simulink model "sampleModel255"  (R2021b)
settings: Solver=VariableStepAuto  StartTime=0.0  StopTime=10.0  RelTol=1e-3
undefined symbols (not defined in the file or in its folder): Newton, Raphson
libraries: simulink x14, slpidlib x3
settings Model: Creator=user  LastModifiedBy=user

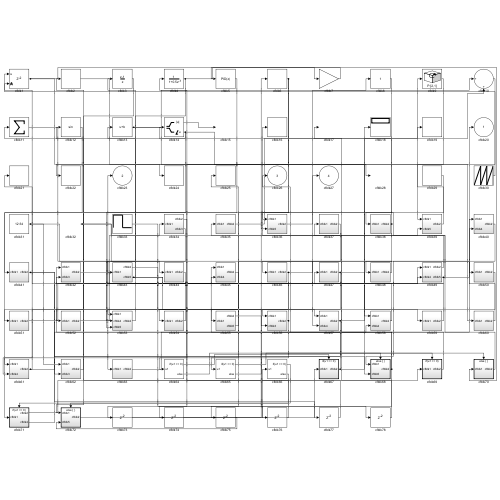
[thumbnail: Simulink's stored preview of the top-level diagram]
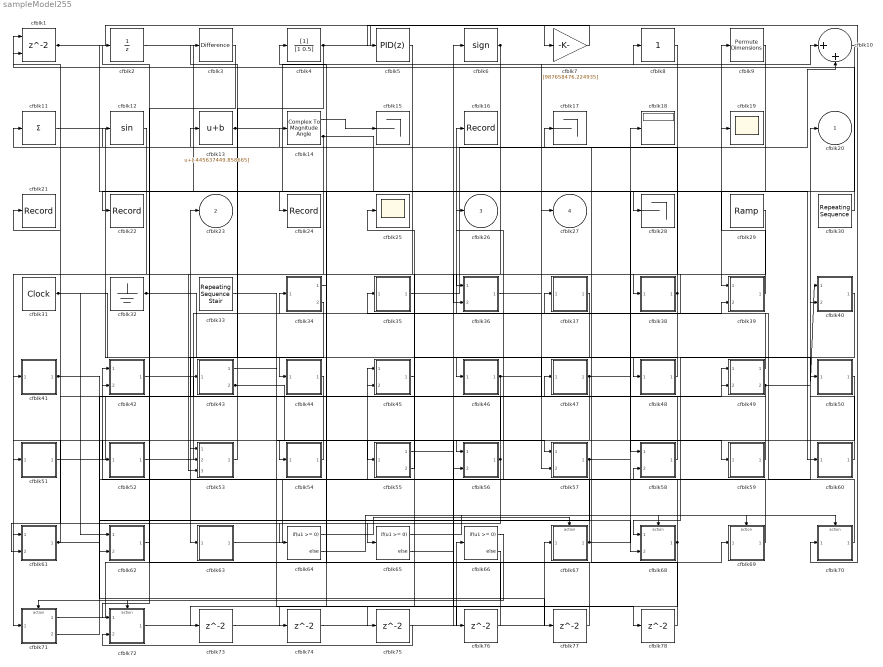
== system sampleModel255 ==
  cfblk1 : Delay  ShowEnablePort=on  SampleTime=1
      settings: InputPortMap=u0,e6
  cfblk10 : Sum  Inputs=|++
  cfblk11 : Sum  Inputs=+
  cfblk12 : Trigonometry
  cfblk13 : Bias  Bias=[-445637449.858665]
  cfblk14 : ComplexToMagnitudeAngle
  cfblk15 : Terminator
  cfblk16 : Record  FileSettingsInternal="{\"entries\":[{\"content\":{\"excelSettings\":{\"content\":{},\"type\":\"Streamout.ExcelSettings\"}},\"type\":\"Streamout.FileSettingStorage\",\"uuid\":\"bcba30e2-a7e8-405a-9570-f6df06466bcb\"}],\"packageUris\":[\"http://schema.mathworks.com/mf0/streamout_blocks/R2020a\"],\"version\":\"1.0\"}"  SignalsInternal="{\"entries\":[{\"content\":{\"signals\":[{\"content\":{\"blockPath\":[\"sampleModel255/cfblk16\"],\"channel\":[],\"dimensions\":[1],\"domain\":\"sampleModel255/cfblk16\",\"lineColor\":\"#a2142f\",\"plots\":[1],\"port\":1,\"sid\":[\"\"],\"signalID\":10495,\"signalName\":\"cfblk49:1\"},\"type\":\"RecordBlkView.Signal\",\"uuid\":\"f066bb72-dd2c-4bd8-bcfc-d20f2ea079be\"}]},\"type\":\"RecordBlkView.InputSignals\",\"uuid\":\"8c248f1a-7e81-44ad-9cf1-3fb42dcd53a2\"}],\"packageUris\":[\"http://schema.mathworks.com/mf0/streamout_blocks/R2020a\"],\"version\":\"1.0\"}"  VisualizationBindings="{\"sparklinesplugin\":{\"info\":[{\"bindingParametersList\":[],\"subplotID\":1}]}}"
  cfblk17 : Terminator
  cfblk18 : Display
  cfblk19 : Scope
  cfblk2 : UnitDelay  HasFrameUpgradeWarning=on
  cfblk21 : Record  FileSettingsInternal="{\"entries\":[{\"content\":{\"excelSettings\":{\"content\":{},\"type\":\"Streamout.ExcelSettings\"}},\"type\":\"Streamout.FileSettingStorage\",\"uuid\":\"b9985514-311d-45c5-af3a-e7c1f733d656\"}],\"packageUris\":[\"http://schema.mathworks.com/mf0/streamout_blocks/R2020a\"],\"version\":\"1.0\"}"  SignalsInternal="{\"entries\":[{\"content\":{\"signals\":[{\"content\":{\"blockPath\":[\"sampleModel255/cfblk21\"],\"channel\":[],\"dimensions\":[1],\"domain\":\"sampleModel255/cfblk21\",\"lineColor\":\"#139fff\",\"plots\":[1],\"port\":1,\"sid\":[\"\"],\"signalID\":10499,\"signalName\":\"cfblk61\"},\"type\":\"RecordBlkView.Signal\",\"uuid\":\"f6652fd2-6723-4bcc-91e8-5e90c24315f7\"}]},\"type\":\"RecordBlkView.InputSignals\",\"uuid\":\"2368f533-53f0-4e7a-ae71-17d9113fb9a7\"}],\"packageUris\":[\"http://schema.mathworks.com/mf0/streamout_blocks/R2020a\"],\"version\":\"1.0\"}"  VisualizationBindings="{\"sparklinesplugin\":{\"info\":[{\"bindingParametersList\":[],\"subplotID\":1}]}}"
  cfblk22 : Record  FileSettingsInternal="{\"entries\":[{\"content\":{\"excelSettings\":{\"content\":{},\"type\":\"Streamout.ExcelSettings\"}},\"type\":\"Streamout.FileSettingStorage\",\"uuid\":\"88f16591-4ce5-46ae-b41e-50627f38fa6a\"}],\"packageUris\":[\"http://schema.mathworks.com/mf0/streamout_blocks/R2020a\"],\"version\":\"1.0\"}"  SignalsInternal="{\"entries\":[{\"content\":{\"signals\":[{\"content\":{\"blockPath\":[\"sampleModel255/cfblk22\"],\"channel\":[],\"dimensions\":[1],\"domain\":\"sampleModel255/cfblk22\",\"lineColor\":\"#ff6929\",\"plots\":[1],\"port\":1,\"sid\":[\"\"],\"signalID\":10503,\"signalName\":\"cfblk6\"},\"type\":\"RecordBlkView.Signal\",\"uuid\":\"f2667ad0-e5eb-4991-95e5-8c16daa194bc\"}]},\"type\":\"RecordBlkView.InputSignals\",\"uuid\":\"a00fef7b-4fdb-41ca-9582-1832ec8d802f\"}],\"packageUris\":[\"http://schema.mathworks.com/mf0/streamout_blocks/R2020a\"],\"version\":\"1.0\"}"  VisualizationBindings="{\"sparklinesplugin\":{\"info\":[{\"bindingParametersList\":[],\"subplotID\":1}]}}"
  cfblk24 : Record  FileSettingsInternal="{\"entries\":[{\"content\":{\"excelSettings\":{\"content\":{},\"type\":\"Streamout.ExcelSettings\"}},\"type\":\"Streamout.FileSettingStorage\",\"uuid\":\"b3a82db9-fc42-4abc-b622-48ca2aee477a\"}],\"packageUris\":[\"http://schema.mathworks.com/mf0/streamout_blocks/R2020a\"],\"version\":\"1.0\"}"  SignalsInternal="{\"entries\":[{\"content\":{\"signals\":[{\"content\":{\"blockPath\":[\"sampleModel255/cfblk24\"],\"channel\":[],\"dimensions\":[1],\"domain\":\"sampleModel255/cfblk24\",\"lineColor\":\"#b746ff\",\"plots\":[1],\"port\":1,\"sid\":[\"\"],\"signalID\":10507,\"signalName\":\"cfblk1\"},\"type\":\"RecordBlkView.Signal\",\"uuid\":\"334ec45f-c396-4067-82da-3699b80d794a\"}]},\"type\":\"RecordBlkView.InputSignals\",\"uuid\":\"c4d4681f-74a4-4c02-baf1-17e94cd38f64\"}],\"packageUris\":[\"http://schema.mathworks.com/mf0/streamout_blocks/R2020a\"],\"version\":\"1.0\"}"  VisualizationBindings="{\"sparklinesplugin\":{\"info\":[{\"bindingParametersList\":[],\"subplotID\":1}]}}"
  cfblk25 : Scope
  cfblk28 : Terminator
  cfblk29 : simulink/Sources/Ramp  slope=[-8268.298690]  start=[21.449295]  InitialOutput=[698761.741317]
  cfblk3 : simulink/Discrete/Difference  ICPrevInput=0.0  OutMin=[]  OutMax=[]  OutDataTypeStr=Inherit: Inherit via back propagation  OutDataType=fixdt(1, 16)  OutScaling=2^-10  DoSatur=off
  cfblk30 : simulink/Sources/Repeating Sequence  rep_seq_t=[0 2]  rep_seq_y=[-542728477.597592, 983773123.631840]
  cfblk31 : DigitalClock
  cfblk32 : Ground
  cfblk33 : simulink/Sources/Repeating Sequence Stair  OutValues=[-766357113.287822, -879833908.730717]  tsamp=-1  OutMin=[]  OutMax=[]  OutDataTypeStr=double  OutputDataTypeScalingMode=double  OutDataType=fixdt(0,8)  ConRadixGroup=Best Precision: Vector-wise  OutScaling=2^-12
  cfblk34 : Subsystem
  cfblk35 : Subsystem
  cfblk36 : Subsystem
  cfblk37 : Subsystem
  cfblk38 : Subsystem
  cfblk39 : Subsystem
  cfblk4 : DiscreteFilter  SampleTime=1
  cfblk40 : Subsystem
  cfblk41 : Subsystem
  cfblk42 : Subsystem
  cfblk43 : Subsystem
  cfblk44 : Subsystem
  cfblk45 : Subsystem
  cfblk46 : Subsystem
  cfblk47 : Subsystem
  cfblk48 : Subsystem
  cfblk49 : Subsystem
  cfblk5 : slpidlib/PID Controller  Controller=PID  Form=Parallel  TimeDomain=Discrete-time  UseExternalTs=off  SampleTime=1  IntegratorMethod=Forward Euler  FilterMethod=Forward Euler  ControllerParametersSource=internal  P=1  I=1  D=0  UseFilter=on  N=100  TunerSelectOption=Transfer Function Based (PID Tuner App)  InitialConditionSource=internal  InitialConditionForIntegrator=0  InitialConditionForFilter=0  DifferentiatorICPrevScaledInput=0  ExternalReset=none  TrackingMode=off  Kt=1  LimitOutput=off  SatLimitsSource=internal  UpperSaturationLimit=inf  LowerSaturationLimit=-inf  LinearizeAsGain=off  AntiWindupMode=none  Kb=1  POutMin=[]  POutMax=[]  IOutMin=[]  IOutMax=[]  DOutMin=[]  DOutMax=[]  NOutMin=[]  NOutMax=[]  SumOutMin=[]  SumOutMax=[]  SaturationOutMin=[]  SaturationOutMax=[]  PParamMin=[]  PParamMax=[]  IParamMin=[]  IParamMax=[]  DParamMin=[]  DParamMax=[]  NParamMin=[]  NParamMax=[]  KbParamMin=[]  KbParamMax=[]  KtParamMin=[]  KtParamMax=[]  KbOutMin=[]  KbOutMax=[]  KtOutMin=[]  KtOutMax=[]  IntegratorOutMin=[]  IntegratorOutMax=[]  FilterOutMin=[]  FilterOutMax=[]  SumI1OutMin=[]  SumI1OutMax=[]  SumI2OutMin=[]  SumI2OutMax=[]  SumI3OutMin=[]  SumI3OutMax=[]  SumI4OutMin=[]  SumI4OutMax=[]  SumDOutMin=[]  SumDOutMax=[]  DifferentiatorOutMin=[]  DifferentiatorOutMax=[]  FilterDiffOutCoefMin=[]  FilterDiffOutCoefMax=[]  ReciprocalOutMin=[]  ReciprocalOutMax=[]  SumDenOutMin=[]  SumDenOutMax=[]  SumNumOutMin=[]  SumNumOutMax=[]  DivideOutMin=[]  DivideOutMax=[]  UdiffTsProdOutMin=[]  UdiffTsProdOutMax=[]  NTsProdOutMin=[]  NTsProdOutMax=[]  UintegralTsProdOutMin=[]  UintegralTsProdOutMax=[]  UngainTsProdOutMin=[]  UngainTsProdOutMax=[]  IntegratorContinuousStateAttributes=''  IntegratorStateMustResolveToSignalObject=off  IntegratorRTWStateStorageClass=Auto  FilterContinuousStateAttributes=''  FilterStateMustResolveToSignalObject=off  FilterRTWStateStorageClass=Auto  ParallelPVariant=InternalParameters  IdealPVariant=Disabled  IVariant=InternalParameters  DVariant=InternalParameters  IntegratorVariant=Discrete  SatVariant=Disabled  AWVariant=Passthrough  PCopyVariant=Disabled  TRVariant=Disabled  FdbkBlocksVariant=Forward  IdealPFdbkVariant=Disabled  SatFdbkVariant=Disabled  DerivativeFilterVariant=ForwardEulerFilter  NVariant=InternalParameters  NCopyVariant=Disabled  FilterICVariant=InternalICsFilter  IntegratorICVariant=InternalICs  ExternalResetVariant=Disabled  TRSumVariant=Passthrough  SumFdbkVariant=Disabled  SumVariant=Sum_PID  TsampFilterVariant=InternalTs  TsampNgainVariant=Passthrough  TsampIntegralVariant=Passthrough  ExternalSaturationOutDataTypeStr=Inherit: Same as second input
  cfblk50 : Subsystem
  cfblk51 : Subsystem
  cfblk52 : Subsystem
  cfblk53 : Subsystem
  cfblk54 : Subsystem
  cfblk55 : Subsystem
  cfblk56 : Subsystem
  cfblk57 : Subsystem
  cfblk58 : Subsystem
  cfblk59 : Subsystem
  cfblk6 : Signum
  cfblk60 : Subsystem
  cfblk61 : Subsystem
  cfblk62 : Subsystem
  cfblk63 : Subsystem
  cfblk64 : If  IfExpression=u1 >= 0  SampleTime=1
  cfblk65 : If  IfExpression=u1 >= 0  SampleTime=1
  cfblk66 : If  IfExpression=u1 >= 0  SampleTime=1
  cfblk67 : Subsystem  TreatAsAtomicUnit=on
  cfblk68 : Subsystem  TreatAsAtomicUnit=on
  cfblk69 : Subsystem  TreatAsAtomicUnit=on
  cfblk7 : Gain  Gain=[987658476.224935]
  cfblk70 : Subsystem  TreatAsAtomicUnit=on
  cfblk71 : Subsystem  TreatAsAtomicUnit=on
  cfblk72 : Subsystem  TreatAsAtomicUnit=on
  cfblk{73..78} (6 alike) : Delay  SampleTime=1
  cfblk8 : simulink/Math Operations/Slider Gain  gain=1  low=0  high=2
  cfblk9 : PermuteDimensions
  cfblk20 : Outport
  cfblk23 : Outport  Port=2
  cfblk26 : Outport  Port=3
  cfblk27 : Outport  Port=4
  wires:
  cfblk67/1(cfblk2) -> cfblk45/1(cfblk1), cfblk19/1
  cfblk31/1 -> cfblk62/1(cfblk1), cfblk44/1(cfblk1)
  cfblk5/1 -> cfblk71/1(cfblk1)
  cfblk38/1(cfblk2) -> cfblk48/1(cfblk1), cfblk14/1
  cfblk71/1(cfblk2) -> cfblk69/1(cfblk1)
  cfblk52/1(cfblk2) -> cfblk34/1(cfblk1)
  cfblk69/1(cfblk2) -> cfblk42/1(cfblk1)
  cfblk59/1(cfblk2) -> cfblk23/1
  cfblk10/1 -> cfblk39/1(cfblk1)
  cfblk46/1(cfblk2) -> cfblk51/1(cfblk1), cfblk50/1(cfblk1)
  cfblk44/1(cfblk2) -> cfblk54/1(cfblk1)
  cfblk70/1(cfblk2) -> cfblk38/1(cfblk1)
  cfblk2/1 -> cfblk58/1(cfblk1)
  cfblk11/1 -> cfblk63/1(cfblk1)
  cfblk61/1(cfblk2) -> cfblk21/1, cfblk58/2(cfblk4)
  cfblk33/1 -> cfblk57/1(cfblk1)
  cfblk6/1 -> cfblk22/1, cfblk36/1(cfblk1), cfblk36/2(cfblk5)
  cfblk4/1 -> cfblk70/1(cfblk1), cfblk43/1(cfblk1)
  cfblk32/1 -> cfblk39/2(cfblk5), cfblk57/2(cfblk4)
  cfblk41/1(cfblk2) -> cfblk68/2(cfblk5), cfblk77/1
  cfblk68/1(cfblk2) -> cfblk17/1, cfblk26/1, cfblk73/1
  cfblk1/1 -> cfblk7/1, cfblk24/1
  cfblk14/1 -> cfblk15/1
  cfblk57/1(cfblk2) -> cfblk18/1, cfblk62/2(cfblk3)
  cfblk14/2 -> cfblk11/1, cfblk60/1(cfblk1), cfblk53/3(cfblk5)
  cfblk51/1(cfblk2) -> cfblk27/1
  cfblk50/1(cfblk2) -> cfblk56/1(cfblk1)
  cfblk60/1(cfblk2) -> cfblk20/1
  cfblk49/1(cfblk2) -> cfblk16/1
  cfblk40/1(cfblk2) -> cfblk68/1(cfblk1)
  cfblk49/2(cfblk5) -> cfblk40/1(cfblk1), cfblk47/1(cfblk1), cfblk35/1(cfblk1)
  cfblk30/1 -> cfblk1/1
  cfblk53/1(cfblk2) -> cfblk13/1
  cfblk13/1 -> cfblk10/1, cfblk28/1
  cfblk3/1 -> cfblk72/1(cfblk1)
  cfblk72/1(cfblk2) -> cfblk6/1
  cfblk47/1(cfblk2) -> cfblk61/1(cfblk1), cfblk59/1(cfblk1)
  cfblk37/1(cfblk2) -> cfblk55/1(cfblk1)
  cfblk71/2(cfblk4) -> cfblk45/2(cfblk4)
  cfblk36/1(cfblk2) -> cfblk8/1
  cfblk7/1 -> cfblk5/1
  cfblk58/1(cfblk2) -> cfblk25/1
  cfblk55/2(cfblk5) -> cfblk42/2(cfblk3)
  cfblk48/1(cfblk2) -> cfblk46/1(cfblk1)
  cfblk62/1(cfblk2) -> cfblk2/1
  cfblk56/1(cfblk2) -> cfblk1/2, cfblk64/1
  cfblk43/2(cfblk5) -> cfblk49/1(cfblk1), cfblk56/2(cfblk3), cfblk3/1
  cfblk29/1 -> cfblk65/1
  cfblk39/1(cfblk2) -> cfblk9/1
  cfblk54/1(cfblk2) -> cfblk53/1(cfblk1)
  cfblk42/1(cfblk2) -> cfblk49/2(cfblk4)
  cfblk34/1(cfblk2) -> cfblk61/2(cfblk4)
  cfblk12/1 -> cfblk41/1(cfblk1)
  cfblk63/1(cfblk2) -> cfblk40/2(cfblk4)
  cfblk35/1(cfblk2) -> cfblk10/2
  cfblk8/1 -> cfblk52/1(cfblk1)
  cfblk34/2(cfblk3) -> cfblk53/2(cfblk4)
  cfblk64/1 -> cfblk67/Action
  cfblk64/2 -> cfblk68/Action
  cfblk65/1 -> cfblk69/Action
  cfblk65/2 -> cfblk70/Action
  cfblk66/1 -> cfblk71/Action
  cfblk66/2 -> cfblk72/Action
  cfblk73/1 -> cfblk66/1
  cfblk9/1 -> cfblk74/1
  cfblk74/1 -> cfblk67/1(cfblk1)
  cfblk45/1(cfblk2) -> cfblk75/1
  cfblk75/1 -> cfblk72/2(cfblk5)
  cfblk43/1(cfblk2) -> cfblk76/1
  cfblk76/1 -> cfblk4/1
  cfblk77/1 -> cfblk12/1
  cfblk55/1(cfblk2) -> cfblk78/1
  cfblk78/1 -> cfblk37/1(cfblk1)

== system sampleModel255/cfblk34 ==
  cfblk1 : Inport
  cfblk2 : Outport
  cfblk3 : Outport  Port=2
  wires:
  cfblk1/1 -> cfblk2/1, cfblk3/1

== system sampleModel255/cfblk35 ==
  cfblk1 : Inport
  cfblk3 : Sqrt  Operator=rSqrt  AlgorithmType=Newton-Raphson  SaturateOnIntegerOverflow=on
  cfblk2 : Outport
  wires:
  cfblk3/1 -> cfblk2/1
  cfblk1/1 -> cfblk3/1

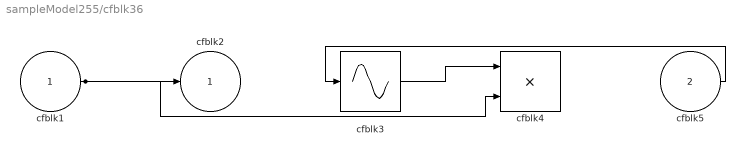
== system sampleModel255/cfblk36 ==
  cfblk1 : Inport
  cfblk5 : Inport  Port=2
  cfblk3 : Sin  TimeSource=Use external signal  SampleTime=0
  cfblk4 : Product  Inputs=**
  cfblk2 : Outport
  wires:
  cfblk1/1 -> cfblk2/1, cfblk4/2
  cfblk3/1 -> cfblk4/1
  cfblk5/1 -> cfblk3/1

== system sampleModel255/cfblk37 ==
  cfblk1 : Inport
  cfblk3 : UnaryMinus
  cfblk4 : Signum
  cfblk2 : Outport
  wires:
  cfblk1/1 -> cfblk3/1
  cfblk3/1 -> cfblk4/1
  cfblk4/1 -> cfblk2/1

== system sampleModel255/cfblk38 ==
  cfblk1 : Inport
  cfblk3 : simulink/Discrete/Transfer Fcn First Order  PoleZ=0.95  ICPrevOutput=0.0  DoSatur=off
  cfblk4 : UnitDelay  HasFrameUpgradeWarning=on
  cfblk2 : Outport
  wires:
  cfblk1/1 -> cfblk3/1
  cfblk4/1 -> cfblk2/1
  cfblk3/1 -> cfblk4/1

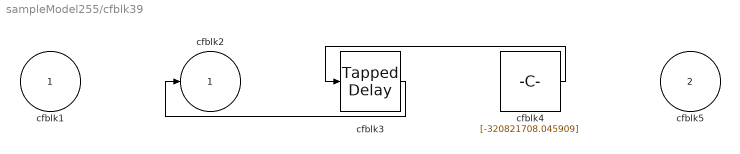
== system sampleModel255/cfblk39 ==
  cfblk1 : Inport
  cfblk5 : Inport  Port=2
  cfblk3 : simulink/Discrete/Tapped Delay  vinit=0.0  samptime=-1  NumDelays=1  DelayOrder=Oldest  includeCurrent=off
  cfblk4 : Constant  Value=[-320821708.045909]  SampleTime=1
  cfblk2 : Outport
  wires:
  cfblk4/1 -> cfblk3/1
  cfblk3/1 -> cfblk2/1

== system sampleModel255/cfblk40 ==
  cfblk1 : Inport
  cfblk4 : Inport  Port=2
  cfblk3 : Constant  Value=[605996582.946135]  SampleTime=1
  cfblk2 : Outport
  wires:
  cfblk4/1 -> cfblk2/1

== system sampleModel255/cfblk41 ==
  cfblk1 : Inport
  cfblk3 : Abs
  cfblk4 : Gain  Gain=[-424041668.466470]
  cfblk2 : Outport
  wires:
  cfblk3/1 -> cfblk2/1
  cfblk1/1 -> cfblk4/1
  cfblk4/1 -> cfblk3/1

== system sampleModel255/cfblk42 ==
  cfblk1 : Inport
  cfblk3 : Inport  Port=2
  cfblk2 : Outport
  wires:
  cfblk1/1 -> cfblk2/1

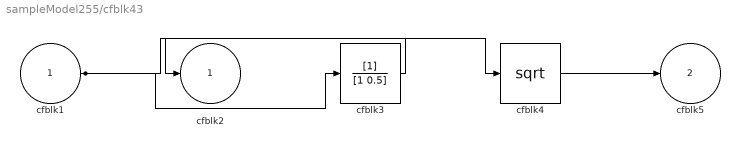
== system sampleModel255/cfblk43 ==
  cfblk1 : Inport
  cfblk3 : DiscreteFilter  SampleTime=1
  cfblk4 : Sqrt  SaturateOnIntegerOverflow=on
  cfblk2 : Outport
  cfblk5 : Outport  Port=2
  wires:
  cfblk3/1 -> cfblk2/1
  cfblk1/1 -> cfblk3/1, cfblk4/1
  cfblk4/1 -> cfblk5/1

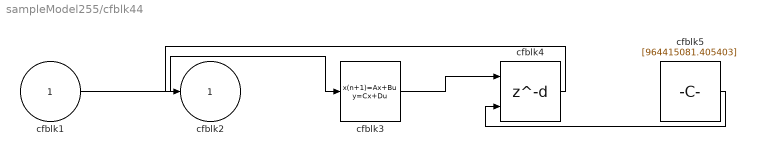
== system sampleModel255/cfblk44 ==
  cfblk1 : Inport
  cfblk3 : DiscreteStateSpace
  cfblk4 : Delay  DelayLengthSource=Input port  SampleTime=1
      settings: InputPortMap=u0,p1
  cfblk5 : Constant  Value=[964415081.405403]  SampleTime=1
  cfblk2 : Outport
  wires:
  cfblk1/1 -> cfblk3/1
  cfblk3/1 -> cfblk4/1
  cfblk5/1 -> cfblk4/2
  cfblk4/1 -> cfblk2/1

== system sampleModel255/cfblk45 ==
  cfblk1 : Inport
  cfblk4 : Inport  Port=2
  cfblk3 : MinMax  Function=max
  cfblk2 : Outport
  wires:
  cfblk3/1 -> cfblk2/1
  cfblk4/1 -> cfblk3/1

== system sampleModel255/cfblk46 ==
  cfblk1 : Inport
  cfblk3 : Trigonometry
  cfblk2 : Outport
  wires:
  cfblk1/1 -> cfblk2/1, cfblk3/1

== system sampleModel255/cfblk47 ==
  cfblk1 : Inport
  cfblk3 : slpidlib/PID Controller  Controller=PID  Form=Parallel  TimeDomain=Discrete-time  UseExternalTs=off  SampleTime=1  IntegratorMethod=Forward Euler  FilterMethod=Forward Euler  ControllerParametersSource=internal  P=1  I=1  D=0  UseFilter=on  N=100  TunerSelectOption=Transfer Function Based (PID Tuner App)  InitialConditionSource=internal  InitialConditionForIntegrator=0  InitialConditionForFilter=0  DifferentiatorICPrevScaledInput=0  ExternalReset=none  TrackingMode=off  Kt=1  LimitOutput=off  SatLimitsSource=internal  UpperSaturationLimit=inf  LowerSaturationLimit=-inf  LinearizeAsGain=off  AntiWindupMode=none  Kb=1  POutMin=[]  POutMax=[]  IOutMin=[]  IOutMax=[]  DOutMin=[]  DOutMax=[]  NOutMin=[]  NOutMax=[]  SumOutMin=[]  SumOutMax=[]  SaturationOutMin=[]  SaturationOutMax=[]  PParamMin=[]  PParamMax=[]  IParamMin=[]  IParamMax=[]  DParamMin=[]  DParamMax=[]  NParamMin=[]  NParamMax=[]  KbParamMin=[]  KbParamMax=[]  KtParamMin=[]  KtParamMax=[]  KbOutMin=[]  KbOutMax=[]  KtOutMin=[]  KtOutMax=[]  IntegratorOutMin=[]  IntegratorOutMax=[]  FilterOutMin=[]  FilterOutMax=[]  SumI1OutMin=[]  SumI1OutMax=[]  SumI2OutMin=[]  SumI2OutMax=[]  SumI3OutMin=[]  SumI3OutMax=[]  SumI4OutMin=[]  SumI4OutMax=[]  SumDOutMin=[]  SumDOutMax=[]  DifferentiatorOutMin=[]  DifferentiatorOutMax=[]  FilterDiffOutCoefMin=[]  FilterDiffOutCoefMax=[]  ReciprocalOutMin=[]  ReciprocalOutMax=[]  SumDenOutMin=[]  SumDenOutMax=[]  SumNumOutMin=[]  SumNumOutMax=[]  DivideOutMin=[]  DivideOutMax=[]  UdiffTsProdOutMin=[]  UdiffTsProdOutMax=[]  NTsProdOutMin=[]  NTsProdOutMax=[]  UintegralTsProdOutMin=[]  UintegralTsProdOutMax=[]  UngainTsProdOutMin=[]  UngainTsProdOutMax=[]  IntegratorContinuousStateAttributes=''  IntegratorStateMustResolveToSignalObject=off  IntegratorRTWStateStorageClass=Auto  FilterContinuousStateAttributes=''  FilterStateMustResolveToSignalObject=off  FilterRTWStateStorageClass=Auto  ParallelPVariant=InternalParameters  IdealPVariant=Disabled  IVariant=InternalParameters  DVariant=InternalParameters  IntegratorVariant=Discrete  SatVariant=Disabled  AWVariant=Passthrough  PCopyVariant=Disabled  TRVariant=Disabled  FdbkBlocksVariant=Forward  IdealPFdbkVariant=Disabled  SatFdbkVariant=Disabled  DerivativeFilterVariant=ForwardEulerFilter  NVariant=InternalParameters  NCopyVariant=Disabled  FilterICVariant=InternalICsFilter  IntegratorICVariant=InternalICs  ExternalResetVariant=Disabled  TRSumVariant=Passthrough  SumFdbkVariant=Disabled  SumVariant=Sum_PID  TsampFilterVariant=InternalTs  TsampNgainVariant=Passthrough  TsampIntegralVariant=Passthrough  ExternalSaturationOutDataTypeStr=Inherit: Same as second input
  cfblk4 : Product
  cfblk5 : Delay  SampleTime=1
  cfblk2 : Outport
  wires:
  cfblk3/1 -> cfblk2/1, cfblk5/1
  cfblk4/1 -> cfblk3/1
  cfblk1/1 -> cfblk4/1
  cfblk5/1 -> cfblk4/2

== system sampleModel255/cfblk48 ==
  cfblk1 : Inport
  cfblk3 : Math  Operator=transpose  SaturateOnIntegerOverflow=on
  cfblk2 : Outport
  wires:
  cfblk1/1 -> cfblk3/1
  cfblk3/1 -> cfblk2/1

== system sampleModel255/cfblk49 ==
  cfblk1 : Inport
  cfblk4 : Inport  Port=2
  cfblk3 : Constant  Value=[-826174241.145449]  SampleTime=1
  cfblk2 : Outport
  cfblk5 : Outport  Port=2
  wires:
  cfblk3/1 -> cfblk5/1
  cfblk4/1 -> cfblk2/1

== system sampleModel255/cfblk50 ==
  cfblk1 : Inport
  cfblk3 : simulink/Discrete/Tapped Delay  vinit=0.0  samptime=-1  NumDelays=1  DelayOrder=Oldest  includeCurrent=off
  cfblk2 : Outport
  wires:
  cfblk1/1 -> cfblk3/1
  cfblk3/1 -> cfblk2/1

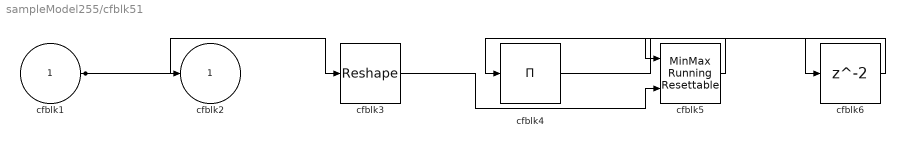
== system sampleModel255/cfblk51 ==
  cfblk1 : Inport
  cfblk3 : Reshape
  cfblk4 : Product  Inputs=*
  cfblk5 : simulink/Math Operations/MinMax Running Resettable  Function=min  vinit=0.0
  cfblk6 : Delay  SampleTime=1
  cfblk2 : Outport
  wires:
  cfblk5/1 -> cfblk4/1
  cfblk1/1 -> cfblk3/1, cfblk2/1
  cfblk3/1 -> cfblk5/2
  cfblk4/1 -> cfblk6/1
  cfblk6/1 -> cfblk5/1

== system sampleModel255/cfblk52 ==
  cfblk1 : Inport
  cfblk3 : simulink/Discrete/Transfer Fcn First Order  PoleZ=0.95  ICPrevOutput=0.0  DoSatur=off
  cfblk2 : Outport
  wires:
  cfblk1/1 -> cfblk3/1
  cfblk3/1 -> cfblk2/1

== system sampleModel255/cfblk53 ==
  cfblk1 : Inport
  cfblk4 : Inport  Port=2
  cfblk5 : Inport  Port=3
  cfblk3 : Sum
  cfblk2 : Outport
  wires:
  cfblk4/1 -> cfblk2/1
  cfblk1/1 -> cfblk3/1
  cfblk5/1 -> cfblk3/2

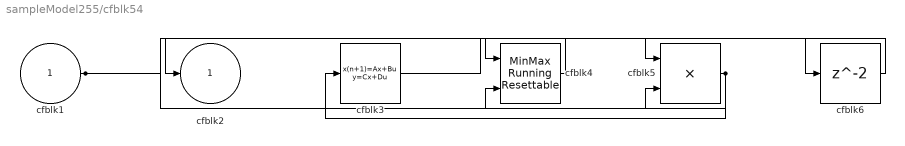
== system sampleModel255/cfblk54 ==
  cfblk1 : Inport
  cfblk3 : DiscreteStateSpace
  cfblk4 : simulink/Math Operations/MinMax Running Resettable  Function=min  vinit=0.0
  cfblk5 : Product  Inputs=**
  cfblk6 : Delay  SampleTime=1
  cfblk2 : Outport
  wires:
  cfblk4/1 -> cfblk2/1
  cfblk1/1 -> cfblk4/1, cfblk5/2
  cfblk5/1 -> cfblk3/1, cfblk4/2
  cfblk3/1 -> cfblk6/1
  cfblk6/1 -> cfblk5/1

== system sampleModel255/cfblk55 ==
  cfblk1 : Inport
  cfblk3 : Rounding
  cfblk4 : simulink/Math Operations/Slider Gain  gain=1  low=0  high=2
  cfblk2 : Outport
  cfblk5 : Outport  Port=2
  wires:
  cfblk3/1 -> cfblk4/1
  cfblk1/1 -> cfblk5/1, cfblk3/1
  cfblk4/1 -> cfblk2/1

== system sampleModel255/cfblk56 ==
  cfblk1 : Inport
  cfblk3 : Inport  Port=2
  cfblk2 : Outport
  wires:
  cfblk1/1 -> cfblk2/1

== system sampleModel255/cfblk57 ==
  cfblk1 : Inport
  cfblk4 : Inport  Port=2
  cfblk3 : Polyval  Coefs=[ +2.081618890e-019, -1.441693666e-014, +4.719686976e-010, -8.536869453e-006, +1.621573104e-001, -8.087801117e+001 ]
  cfblk2 : Outport
  wires:
  cfblk1/1 -> cfblk2/1
  cfblk4/1 -> cfblk3/1

== system sampleModel255/cfblk58 ==
  cfblk1 : Inport
  cfblk4 : Inport  Port=2
  cfblk3 : ComplexToRealImag
  cfblk2 : Outport
  wires:
  cfblk1/1 -> cfblk2/1
  cfblk4/1 -> cfblk3/1

== system sampleModel255/cfblk59 ==
  cfblk1 : Inport
  cfblk3 : Sqrt  SaturateOnIntegerOverflow=on
  cfblk4 : Signum
  cfblk5 : UnaryMinus
  cfblk2 : Outport
  wires:
  cfblk3/1 -> cfblk4/1
  cfblk1/1 -> cfblk3/1
  cfblk4/1 -> cfblk5/1
  cfblk5/1 -> cfblk2/1

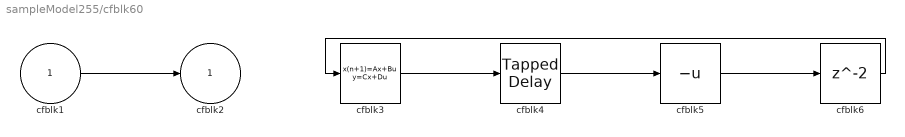
== system sampleModel255/cfblk60 ==
  cfblk1 : Inport
  cfblk3 : DiscreteStateSpace
  cfblk4 : simulink/Discrete/Tapped Delay  vinit=0.0  samptime=-1  NumDelays=1  DelayOrder=Oldest  includeCurrent=off
  cfblk5 : UnaryMinus
  cfblk6 : Delay  SampleTime=1
  cfblk2 : Outport
  wires:
  cfblk4/1 -> cfblk5/1
  cfblk1/1 -> cfblk2/1
  cfblk3/1 -> cfblk4/1
  cfblk5/1 -> cfblk6/1
  cfblk6/1 -> cfblk3/1

== system sampleModel255/cfblk61 ==
  cfblk1 : Inport
  cfblk4 : Inport  Port=2
  cfblk3 : Constant  Value=[-689178807.138897]  SampleTime=1
  cfblk2 : Outport
  wires:
  cfblk3/1 -> cfblk2/1

== system sampleModel255/cfblk62 ==
  cfblk1 : Inport
  cfblk3 : Inport  Port=2
  cfblk2 : Outport
  wires:
  cfblk1/1 -> cfblk2/1

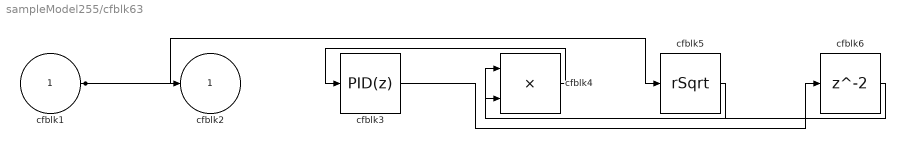
== system sampleModel255/cfblk63 ==
  cfblk1 : Inport
  cfblk3 : slpidlib/PID Controller  Controller=PID  Form=Parallel  TimeDomain=Discrete-time  UseExternalTs=off  SampleTime=1  IntegratorMethod=Forward Euler  FilterMethod=Forward Euler  ControllerParametersSource=internal  P=1  I=1  D=0  UseFilter=on  N=100  TunerSelectOption=Transfer Function Based (PID Tuner App)  InitialConditionSource=internal  InitialConditionForIntegrator=0  InitialConditionForFilter=0  DifferentiatorICPrevScaledInput=0  ExternalReset=none  TrackingMode=off  Kt=1  LimitOutput=off  SatLimitsSource=internal  UpperSaturationLimit=inf  LowerSaturationLimit=-inf  LinearizeAsGain=off  AntiWindupMode=none  Kb=1  POutMin=[]  POutMax=[]  IOutMin=[]  IOutMax=[]  DOutMin=[]  DOutMax=[]  NOutMin=[]  NOutMax=[]  SumOutMin=[]  SumOutMax=[]  SaturationOutMin=[]  SaturationOutMax=[]  PParamMin=[]  PParamMax=[]  IParamMin=[]  IParamMax=[]  DParamMin=[]  DParamMax=[]  NParamMin=[]  NParamMax=[]  KbParamMin=[]  KbParamMax=[]  KtParamMin=[]  KtParamMax=[]  KbOutMin=[]  KbOutMax=[]  KtOutMin=[]  KtOutMax=[]  IntegratorOutMin=[]  IntegratorOutMax=[]  FilterOutMin=[]  FilterOutMax=[]  SumI1OutMin=[]  SumI1OutMax=[]  SumI2OutMin=[]  SumI2OutMax=[]  SumI3OutMin=[]  SumI3OutMax=[]  SumI4OutMin=[]  SumI4OutMax=[]  SumDOutMin=[]  SumDOutMax=[]  DifferentiatorOutMin=[]  DifferentiatorOutMax=[]  FilterDiffOutCoefMin=[]  FilterDiffOutCoefMax=[]  ReciprocalOutMin=[]  ReciprocalOutMax=[]  SumDenOutMin=[]  SumDenOutMax=[]  SumNumOutMin=[]  SumNumOutMax=[]  DivideOutMin=[]  DivideOutMax=[]  UdiffTsProdOutMin=[]  UdiffTsProdOutMax=[]  NTsProdOutMin=[]  NTsProdOutMax=[]  UintegralTsProdOutMin=[]  UintegralTsProdOutMax=[]  UngainTsProdOutMin=[]  UngainTsProdOutMax=[]  IntegratorContinuousStateAttributes=''  IntegratorStateMustResolveToSignalObject=off  IntegratorRTWStateStorageClass=Auto  FilterContinuousStateAttributes=''  FilterStateMustResolveToSignalObject=off  FilterRTWStateStorageClass=Auto  ParallelPVariant=InternalParameters  IdealPVariant=Disabled  IVariant=InternalParameters  DVariant=InternalParameters  IntegratorVariant=Discrete  SatVariant=Disabled  AWVariant=Passthrough  PCopyVariant=Disabled  TRVariant=Disabled  FdbkBlocksVariant=Forward  IdealPFdbkVariant=Disabled  SatFdbkVariant=Disabled  DerivativeFilterVariant=ForwardEulerFilter  NVariant=InternalParameters  NCopyVariant=Disabled  FilterICVariant=InternalICsFilter  IntegratorICVariant=InternalICs  ExternalResetVariant=Disabled  TRSumVariant=Passthrough  SumFdbkVariant=Disabled  SumVariant=Sum_PID  TsampFilterVariant=InternalTs  TsampNgainVariant=Passthrough  TsampIntegralVariant=Passthrough  ExternalSaturationOutDataTypeStr=Inherit: Same as second input
  cfblk4 : Product
  cfblk5 : Sqrt  Operator=rSqrt  AlgorithmType=Newton-Raphson  SaturateOnIntegerOverflow=on
  cfblk6 : Delay  SampleTime=1
  cfblk2 : Outport
  wires:
  cfblk4/1 -> cfblk3/1
  cfblk5/1 -> cfblk4/1
  cfblk1/1 -> cfblk5/1, cfblk2/1
  cfblk3/1 -> cfblk6/1
  cfblk6/1 -> cfblk4/2

== system sampleModel255/cfblk67 ==
  cfblk1 : Inport
  Action Port : ActionPort  ActionPortLabel=if(u1 >= 0)
  cfblk3 : Constant  Value=[457340937.713665]  SampleTime=1
  cfblk4 : Constant  Value=[-182122357.570016]  SampleTime=1
  cfblk2 : Outport
  wires:
  cfblk1/1 -> cfblk2/1

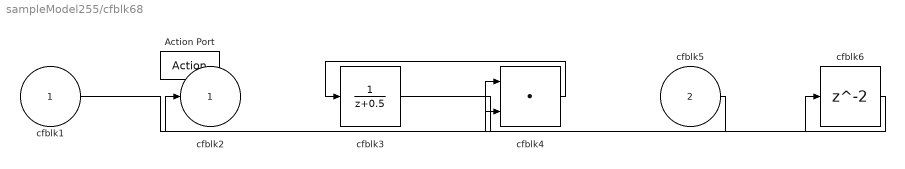
== system sampleModel255/cfblk68 ==
  cfblk1 : Inport
  cfblk5 : Inport  Port=2
  Action Port : ActionPort  ActionPortLabel=else
  cfblk3 : DiscreteTransferFcn
  cfblk4 : DotProduct  InputSameDT=on  OutDataTypeStr=Inherit: Inherit via internal rule
  cfblk6 : Delay
  cfblk2 : Outport
  wires:
  cfblk5/1 -> cfblk2/1
  cfblk4/1 -> cfblk3/1
  cfblk1/1 -> cfblk4/1
  cfblk3/1 -> cfblk6/1
  cfblk6/1 -> cfblk4/2

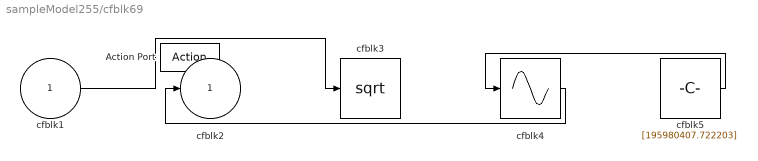
== system sampleModel255/cfblk69 ==
  cfblk1 : Inport
  Action Port : ActionPort  ActionPortLabel=if(u1 >= 0)
  cfblk3 : Sqrt  SaturateOnIntegerOverflow=on
  cfblk4 : Sin  TimeSource=Use external signal  SampleTime=0
  cfblk5 : Constant  Value=[195980407.722203]  SampleTime=1
  cfblk2 : Outport
  wires:
  cfblk5/1 -> cfblk4/1
  cfblk4/1 -> cfblk2/1
  cfblk1/1 -> cfblk3/1

== system sampleModel255/cfblk70 ==
  cfblk1 : Inport
  Action Port : ActionPort  ActionPortLabel=else
  cfblk3 : Sum  Inputs=--
  cfblk4 : Constant  Value=[848109875.902462]  SampleTime=1
  cfblk2 : Outport
  wires:
  cfblk4/1 -> cfblk3/1
  cfblk1/1 -> cfblk2/1, cfblk3/2

== system sampleModel255/cfblk71 ==
  cfblk1 : Inport
  Action Port : ActionPort  ActionPortLabel=if(u1 >= 0)
  cfblk3 : Constant  Value=[-720925123.632533]  SampleTime=1
  cfblk2 : Outport
  cfblk4 : Outport  Port=2
  wires:
  cfblk1/1 -> cfblk2/1
  cfblk3/1 -> cfblk4/1

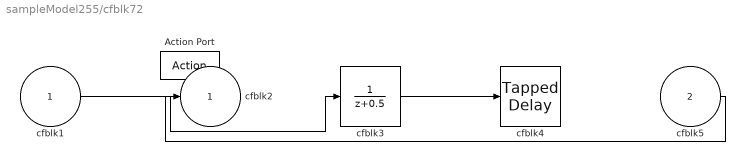
== system sampleModel255/cfblk72 ==
  cfblk1 : Inport
  cfblk5 : Inport  Port=2
  Action Port : ActionPort  ActionPortLabel=else
  cfblk3 : DiscreteTransferFcn
  cfblk4 : simulink/Discrete/Tapped Delay  vinit=0.0  samptime=-1  NumDelays=1  DelayOrder=Oldest  includeCurrent=off
  cfblk2 : Outport
  wires:
  cfblk3/1 -> cfblk4/1
  cfblk1/1 -> cfblk3/1
  cfblk5/1 -> cfblk2/1
